simulink model "Zadanie_3"  (Simulink 7.1)
settings: Solver=ode45  StartTime=0.0  StopTime=4  RelTol=1e-3
settings Model: Creator=Michal  LastModifiedBy=Michal

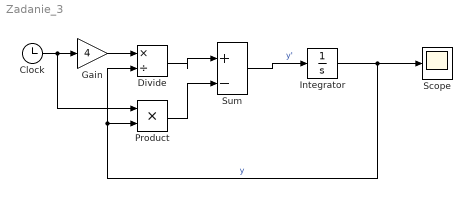
== system Zadanie_3 ==
  Clock : Clock
      settings: Decimation=10
  Divide : Product  Inputs=*/  OutDataType=sfix(16)  OutScaling=2^-10
  Gain : Gain  Gain=4  ParameterDataType=sfix(16)  ParameterScaling=2^0  OutDataType=sfix(16)  OutScaling=2^0
  Integrator : Integrator  InitialCondition=1
  Product : Product  OutDataType=sfix(16)  OutScaling=2^0  RndMeth=Zero
  Scope : Scope
  Sum : Sum  Inputs=|+-  OutDataType=sfix(16)  OutScaling=2^0
  wires:
  Clock/1 -> Gain/1, Product/1
  Integrator/1 -> Scope/1, Divide/2, Product/2  "y"
  Gain/1 -> Divide/1
  Product/1 -> Sum/2
  Sum/1 -> Integrator/1  "y'"
  Divide/1 -> Sum/1
